simulink model "ode2"  (Simulink 8.0)
settings: Solver=ode4  StartTime=0.0  StopTime=10.0  FixedStep=0.01  RelTol=1e-3
libraries: simulink x1
settings Model: Creator=CAD  LastModifiedBy=CAD

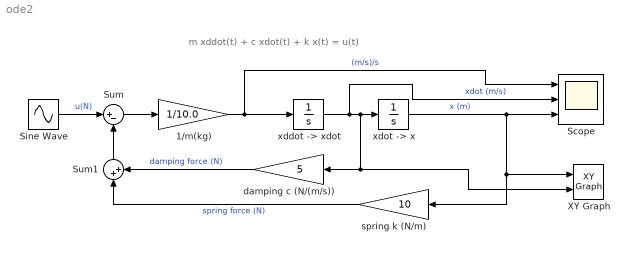
== system ode2 ==
  note: m xddot(t) + c xdot(t) + k x(t) = u(t)
  1/m(kg) : Gain  Gain=1/10.0
  Scope : Scope  NumInputPorts=3
      settings: TimeRange=10  YMin=-6~-4~-4  YMax=4~2~6
  Sine Wave : Sin  Amplitude=0  SampleTime=0
  Sum : Sum  Inputs=|+-
  Sum1 : Sum  Inputs=|++
  XY Graph : simulink/Sinks/XY Graph  xmin=-7  xmax=7  ymin=-6  ymax=6  st=-1
  damping c (N/(m/s)) : Gain  Gain=5
  spring k (N/m) : Gain  Gain=10
  "xddot -> xdot" : Integrator
  "xdot -> x" : Integrator  InitialCondition=5
  wires:
  "xdot -> x"/1 -> XY Graph/1, spring k (N/m)/1, Scope/3  "x (m)"
  "xddot -> xdot"/1 -> Scope/2, damping c (N/(m/s))/1, XY Graph/2, "xdot -> x"/1  "xdot (m/s)"
  1/m(kg)/1 -> Scope/1, "xddot -> xdot"/1  "(m/s)/s"
  spring k (N/m)/1 -> Sum1/1  "spring force (N)"
  damping c (N/(m/s))/1 -> Sum1/2  "damping force (N)"
  Sum/1 -> 1/m(kg)/1
  Sine Wave/1 -> Sum/1  "u(N)"
  Sum1/1 -> Sum/2
